simulink model "sampleModel2037_4_sub"  (R2023a)
settings: Solver=VariableStepAuto  StartTime=0.0  StopTime=10.0  RelTol=1e-3
libraries: hdlsllib x5
settings Model: Creator=user1  LastModifiedBy=user1

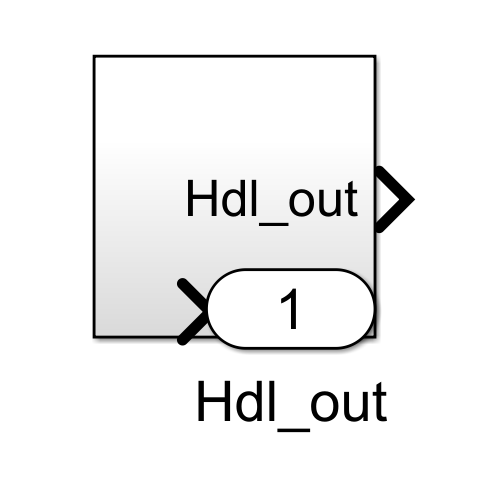
[thumbnail: Simulink's stored preview of the top-level diagram]
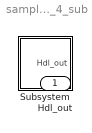
== system sampleModel2037_4_sub ==
  Subsystem : Subsystem
  Hdl_out : Outport  OutDataTypeStr=uint8

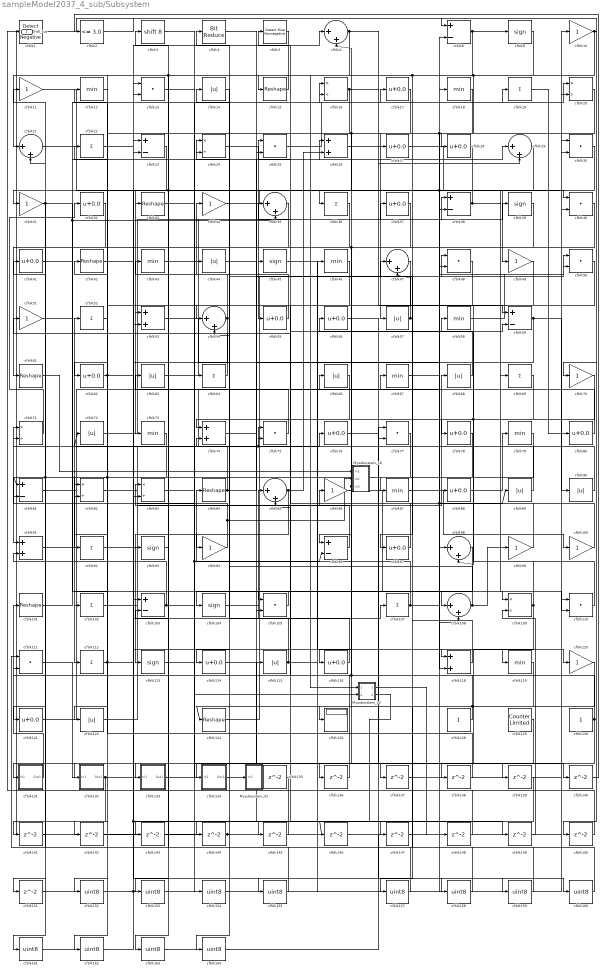
== system sampleModel2037_4_sub/Subsystem ==
  Mysubsystem_18 : Subsystem  TreatAsAtomicUnit=on  RTWFcnName=Mysubsystem_18
      settings: RTWFcnNameOpts=User specified  RTWFileNameOpts=Use function name
  Mysubsystem_20 : Subsystem  TreatAsAtomicUnit=on  RTWFcnName=Mysubsystem_20
      settings: RTWFcnNameOpts=User specified  RTWFileNameOpts=Use function name
  Mysubsystem_31 : Subsystem  TreatAsAtomicUnit=on  RTWFcnName=Mysubsystem_31
      settings: RTWFcnNameOpts=User specified  RTWFileNameOpts=Use function name
  cfblk1 : hdlsllib/Logic and Bit Operations/Detect Fall Negative  vinit=0  OutDataTypeStr=uint8
  cfblk{10..11,31,34,49,51,70,86,94,99..100,120} (12 alike) : Gain  OutDataTypeStr=uint8
  cfblk{15,33,42,61,84,101,124} (7 alike) : Reshape
  cfblk{19,22,36,52,64,69,92,102,107,112} (10 alike) : Sum  Inputs=+  OutDataTypeStr=uint8
  cfblk{8,23,38,59,81,96,103} (7 alike) : Sum  Inputs=+-  OutDataTypeStr=uint8
  cfblk{9,39,45,93,104,113} (6 alike) : Signum
  cfblk{13,25,30,40,48,50,75,77,105,110..111} (11 alike) : DotProduct  OutDataTypeStr=uint8
  cfblk{6,21,29,35,47,54,85,98,108} (9 alike) : Sum  Inputs=|++  OutDataTypeStr=uint8
  cfblk{16,20,24,71,82..83,109} (7 alike) : Product  Inputs=*/  OutDataTypeStr=uint8  RndMeth=Zero  SaturateOnIntegerOverflow=on
  cfblk{17,27..28,32,37,41,55..56,62,76,78,80,88,97,114,116,121} (17 alike) : Bias  Bias=0.0  SaturateOnIntegerOverflow=off
  cfblk{14,44,57,63,66,68,72,89..90,115,122} (11 alike) : Abs  OutDataTypeStr=uint8  SaturateOnIntegerOverflow=off
  cfblk{26,53,74,91,118} (5 alike) : Sum  OutDataTypeStr=uint8
  cfblk{12,18,43,46,58,67,73,79,87,119} (10 alike) : MinMax  OutDataTypeStr=uint8
  cfblk126 : Display
  cfblk128 : Constant  OutDataTypeStr=uint8  SampleTime=-1
  cfblk129 : hdlsllib/Sources/Counter Limited  uplimit=7  tsamp=-1
  cfblk130 : Constant  OutDataTypeStr=uint8  SampleTime=-1
  cfblk131 : Subsystem
      settings: LibrarySourceBlock=|
      | hdlsllib/Ports &
      | Subsystems/Subsystem
  cfblk132 : Subsystem
      settings: LibrarySourceBlock=|
      | hdlsllib/Ports &
      | Subsystems/Subsystem
  cfblk133 : Subsystem
      settings: LibrarySourceBlock=|
      | hdlsllib/Ports &
      | Subsystems/Subsystem
  cfblk134 : Subsystem
      settings: LibrarySourceBlock=|
      | hdlsllib/Ports &
      | Subsystems/Subsystem
  cfblk{135..151} (17 alike) : Delay  SampleTime=1
  cfblk{152..155,157..164} (12 alike) : DataTypeConversion  OutDataTypeStr=uint8  SaturateOnIntegerOverflow=off  RndMeth=Floor
  cfblk2 : hdlsllib/Logic and Bit Operations/Compare To Constant  relop=<=  const=3.0  OutDataTypeStr=uint8
  cfblk3 : ArithShift  BitShiftNumber=8
  cfblk4 : hdlsllib/Logic and Bit Operations/Bit Reduce  mode=AND
  cfblk5 : hdlsllib/Logic and Bit Operations/Detect Rise Nonnegative  vinit=0  OutDataTypeStr=uint8
  Hdl_out : Outport  OutDataTypeStr=uint8
  wires:
  cfblk105/1 -> cfblk104/1
  cfblk72/1 -> cfblk38/1
  cfblk122/1 -> cfblk86/1
  cfblk11/1 -> cfblk49/1
  cfblk36/1 -> cfblk61/1
  cfblk17/1 -> cfblk57/1
  cfblk19/1 -> cfblk80/1
  cfblk63/1 -> cfblk37/1
  cfblk66/1 -> cfblk134/1(In1)
  cfblk71/1 -> cfblk32/1
  cfblk23/1 -> cfblk73/1
  cfblk131/1(Out1) -> cfblk101/1
  cfblk108/1 -> cfblk54/2, cfblk99/1
  cfblk121/1 -> cfblk66/1
  cfblk112/1 -> cfblk118/1, cfblk12/1
  cfblk43/1 -> cfblk39/1
  cfblk15/1 -> cfblk21/1
  cfblk104/1 -> cfblk76/1
  cfblk99/1 -> cfblk51/1
  cfblk97/1 -> cfblk5/1
  cfblk98/1 -> cfblk114/1
  cfblk79/1 -> cfblk112/1
  cfblk124/1 -> cfblk50/1
  cfblk114/1 -> cfblk119/1
  cfblk90/1 -> cfblk56/1
  cfblk100/1 -> cfblk68/1
  cfblk70/1 -> cfblk74/1
  cfblk26/1 -> cfblk27/1
  cfblk69/1 -> cfblk98/2, Mysubsystem_18/3(In3), cfblk126/1
  cfblk93/1 -> cfblk133/1(In1)
  cfblk27/1 -> cfblk69/1
  cfblk116/1 -> cfblk24/1
  cfblk49/1 -> cfblk78/1
  cfblk1/1 -> cfblk70/1
  cfblk91/1 -> cfblk52/1
  cfblk42/1 -> cfblk155/1, cfblk146/1
  cfblk118/1 -> cfblk47/1
  cfblk86/1 -> cfblk109/1
  cfblk18/1 -> cfblk118/2, cfblk62/1
  cfblk134/1(Out1) -> cfblk115/1
  cfblk55/1 -> cfblk34/1
  cfblk81/1 -> cfblk18/1
  cfblk89/1 -> cfblk14/1
  cfblk38/1 -> cfblk110/2, cfblk31/1
  cfblk24/1 -> cfblk55/1
  cfblk6/1 -> cfblk59/1, cfblk15/1
  cfblk34/1 -> cfblk40/1
  cfblk80/1 -> cfblk25/1
  cfblk94/1 -> cfblk71/1, Mysubsystem_18/2(In2)
  cfblk85/1 -> cfblk26/2, cfblk113/1
  cfblk110/1 -> cfblk58/1
  cfblk133/1(Out1) -> cfblk96/2, cfblk20/1
  cfblk5/1 -> cfblk102/1
  cfblk109/1 -> cfblk138/1, cfblk72/1, cfblk75/1
  cfblk54/1 -> cfblk83/2, cfblk43/1
  cfblk2/1 -> cfblk8/1
  cfblk64/1 -> cfblk42/1
  cfblk87/1 -> cfblk100/1
  cfblk57/1 -> cfblk4/1, cfblk97/1
  cfblk92/1 -> cfblk74/2
  cfblk30/1 -> cfblk45/1
  cfblk47/1 -> cfblk116/1
  cfblk107/1 -> cfblk84/1, cfblk50/2, cfblk89/1
  cfblk46/1 -> cfblk152/1
  cfblk35/1 -> cfblk122/1
  cfblk20/1 -> cfblk36/1, cfblk94/1
  cfblk21/1 -> cfblk24/2
  cfblk9/1 -> cfblk28/1, cfblk25/2, cfblk47/2
  cfblk25/1 -> cfblk17/1
  cfblk128/1 -> cfblk124/1, cfblk6/2, cfblk85/2
  cfblk82/1 -> cfblk44/1
  cfblk62/1 -> cfblk92/1, cfblk23/2
  cfblk88/1 -> cfblk79/1
  cfblk130/1 -> cfblk131/1(In1), cfblk41/1
  cfblk40/1 -> cfblk136/1, cfblk54/1
  cfblk113/1 -> cfblk75/2
  cfblk115/1 -> cfblk59/2, cfblk85/1
  cfblk96/1 -> cfblk83/1
  cfblk132/1(Out1) -> cfblk161/1, cfblk107/1
  cfblk73/1 -> cfblk91/1
  cfblk12/1 -> cfblk82/1
  cfblk78/1 -> cfblk142/1, cfblk141/1
  cfblk103/1 -> cfblk81/2, cfblk88/1
  cfblk59/1 -> cfblk105/2, cfblk90/1
  cfblk102/1 -> cfblk64/1
  cfblk22/1 -> cfblk6/1
  cfblk45/1 -> cfblk120/1
  cfblk68/1 -> cfblk35/1
  cfblk44/1 -> cfblk108/1
  cfblk32/1 -> cfblk151/1, cfblk81/1
  cfblk84/1 -> cfblk29/1, cfblk11/1
  cfblk101/1 -> cfblk26/1
  cfblk10/1 -> cfblk150/1, cfblk33/1, cfblk132/1(In1)
  cfblk39/1 -> cfblk87/1
  cfblk31/1 -> cfblk121/1, cfblk105/1
  cfblk67/1 -> cfblk19/1
  cfblk52/1 -> cfblk22/1
  cfblk58/1 -> cfblk10/1
  cfblk53/1 -> cfblk98/1
  cfblk75/1 -> cfblk63/1
  cfblk41/1 -> cfblk16/2, cfblk35/2
  cfblk74/1 -> cfblk48/1
  cfblk8/1 -> cfblk9/1, Mysubsystem_20/1(In1)
  cfblk51/1 -> cfblk16/1
  cfblk16/1 -> cfblk29/2, cfblk93/1
  cfblk37/1 -> cfblk96/1
  cfblk50/1 -> cfblk53/1
  cfblk29/1 -> cfblk48/2, cfblk143/1, cfblk53/2
  cfblk48/1 -> cfblk135/1
  cfblk135/1 -> cfblk1/1
  cfblk136/1 -> cfblk71/2
  cfblk83/1 -> cfblk137/1
  cfblk137/1 -> cfblk40/2
  cfblk138/1 -> cfblk82/2
  cfblk76/1 -> cfblk139/1
  cfblk56/1 -> cfblk140/1
  cfblk140/1 -> cfblk2/1
  cfblk141/1 -> cfblk21/2
  cfblk142/1 -> cfblk20/2
  cfblk143/1 -> cfblk110/1
  cfblk14/1 -> cfblk144/1
  cfblk144/1 -> Hdl_out/1, cfblk38/2
  cfblk120/1 -> cfblk145/1
  cfblk145/1 -> cfblk91/2
  cfblk4/1 -> cfblk147/1
  cfblk147/1 -> cfblk8/2
  cfblk148/1 -> cfblk23/1
  cfblk149/1 -> cfblk109/2
  cfblk150/1 -> cfblk103/2
  cfblk151/1 -> cfblk108/2
  cfblk152/1 -> cfblk158/1, cfblk30/2
  cfblk129/1 -> cfblk153/1
  cfblk153/1 -> cfblk46/1
  cfblk3/1 -> cfblk154/1
  cfblk154/1 -> cfblk30/1
  cfblk155/1 -> cfblk3/1
  cfblk119/1 -> cfblk157/1
  cfblk157/1 -> cfblk111/1
  cfblk158/1 -> cfblk111/2
  cfblk13/1 -> cfblk159/1
  cfblk159/1 -> cfblk67/1
  cfblk146/1 -> cfblk160/1
  cfblk160/1 -> cfblk13/1
  cfblk161/1 -> cfblk13/2
  cfblk77/1 -> cfblk162/1
  cfblk162/1 -> cfblk103/1
  cfblk139/1 -> cfblk163/1
  cfblk163/1 -> cfblk77/1
  cfblk28/1 -> cfblk164/1
  cfblk164/1 -> cfblk77/2
  cfblk61/1 -> Mysubsystem_18/1(In1)
  cfblk33/1 -> Mysubsystem_20/2(In2)
  Mysubsystem_20/1(Out1) -> cfblk148/1
  Mysubsystem_20/2(Out2) -> cfblk149/1
  cfblk111/1 -> Mysubsystem_31/1(In1)

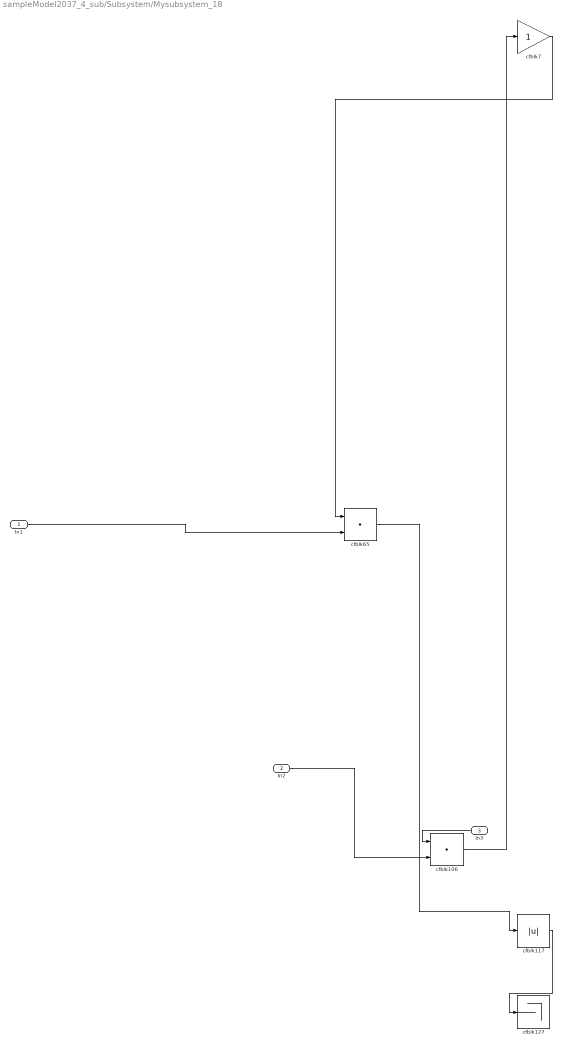
== system sampleModel2037_4_sub/Subsystem/Mysubsystem_18 ==
  In1 : Inport
  In2 : Inport  Port=2
  In3 : Inport  Port=3
  cfblk106 : DotProduct  OutDataTypeStr=Inherit: Inherit via internal rule
  cfblk117 : Abs  SaturateOnIntegerOverflow=off
  cfblk127 : Terminator
  cfblk65 : DotProduct  OutDataTypeStr=Inherit: Inherit via internal rule
  cfblk7 : Gain
  wires:
  In2/1 -> cfblk106/2
  cfblk106/1 -> cfblk7/1
  cfblk65/1 -> cfblk117/1
  cfblk117/1 -> cfblk127/1
  In3/1 -> cfblk106/1
  In1/1 -> cfblk65/2
  cfblk7/1 -> cfblk65/1

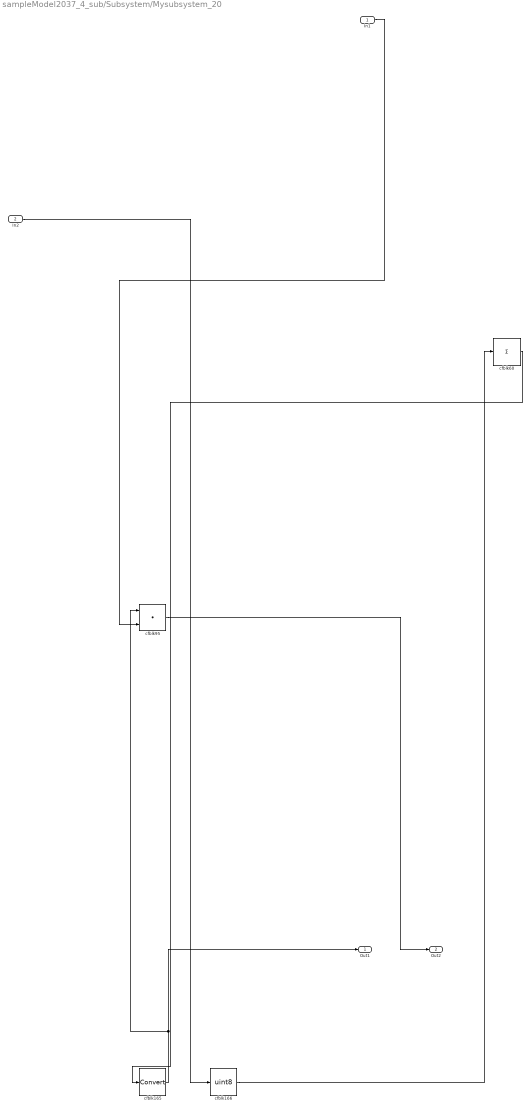
== system sampleModel2037_4_sub/Subsystem/Mysubsystem_20 ==
  In1 : Inport
  In2 : Inport  Port=2
  cfblk165 : DataTypeConversion  SaturateOnIntegerOverflow=off  RndMeth=Floor
  cfblk166 : DataTypeConversion  OutDataTypeStr=uint8  SaturateOnIntegerOverflow=off  RndMeth=Floor
  cfblk60 : Sum  Inputs=+
  cfblk95 : DotProduct  OutDataTypeStr=Inherit: Inherit via internal rule
  Out1 : Outport
  Out2 : Outport  Port=2
  wires:
  In1/1 -> cfblk95/2
  cfblk166/1 -> cfblk60/1
  cfblk95/1 -> Out2/1
  In2/1 -> cfblk166/1
  cfblk165/1 -> cfblk95/1, Out1/1
  cfblk60/1 -> cfblk165/1

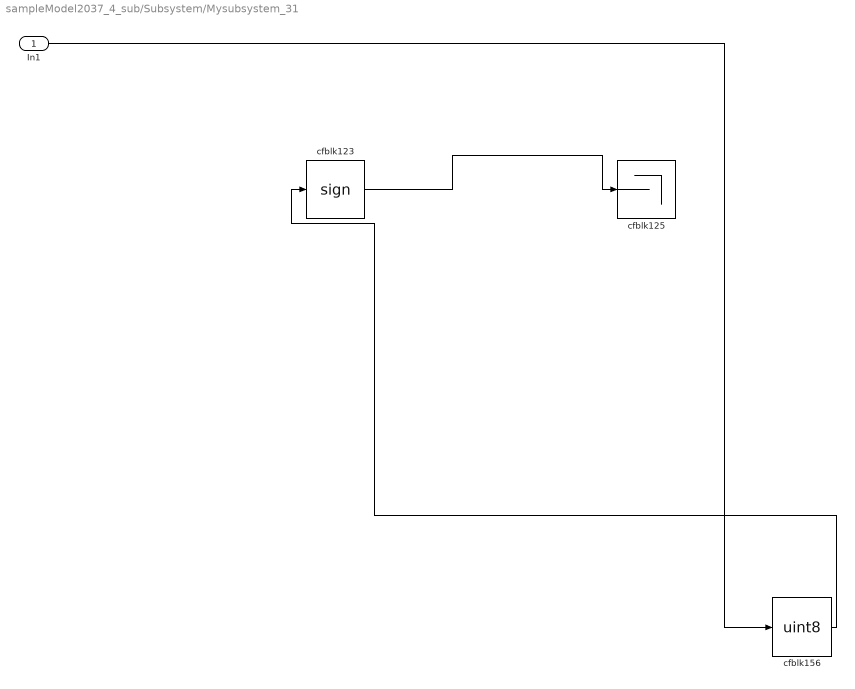
== system sampleModel2037_4_sub/Subsystem/Mysubsystem_31 ==
  In1 : Inport
  cfblk123 : Signum
  cfblk125 : Terminator
  cfblk156 : DataTypeConversion  OutDataTypeStr=uint8  SaturateOnIntegerOverflow=off  RndMeth=Floor
  wires:
  In1/1 -> cfblk156/1
  cfblk156/1 -> cfblk123/1
  cfblk123/1 -> cfblk125/1

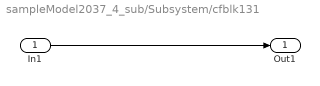
== system sampleModel2037_4_sub/Subsystem/cfblk131 ==
  In1 : Inport
  Out1 : Outport
  wires:
  In1/1 -> Out1/1

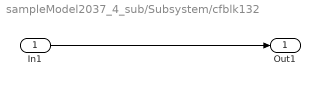
== system sampleModel2037_4_sub/Subsystem/cfblk132 ==
  In1 : Inport
  Out1 : Outport
  wires:
  In1/1 -> Out1/1

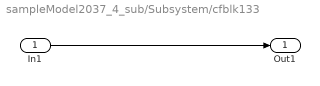
== system sampleModel2037_4_sub/Subsystem/cfblk133 ==
  In1 : Inport
  Out1 : Outport
  wires:
  In1/1 -> Out1/1

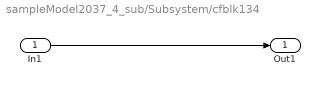
== system sampleModel2037_4_sub/Subsystem/cfblk134 ==
  In1 : Inport
  Out1 : Outport
  wires:
  In1/1 -> Out1/1
